simulink library "se2a_environment_lib"  (R2018b)
settings: Solver=VariableStepAuto  StartTime=0.0  StopTime=10.0  RelTol=1e-3
undefined symbols (not defined in the file or in its folder): aircraft, alt_ground, atmosphere, Atmosphere, cntrl, envir, g, ic, pos_ref, wind
libraries: simulink x9, atmosphere_lib x6, linear_systems_lib x6, $bdroot x5
(part 2 of 2)

== system se2a_environment_lib/Environment with Lidar WindEst/wind at wings1/Sort_TrueWind_Wing ==
  True_Wind_Sec : Inport
  Matrix Concatenate : Concatenate  NumInputs=3  Mode=Multidimensional array
  Matrix Concatenate1 : Concatenate  NumInputs=3  Mode=Multidimensional array
  Reshape{,1..5} (6 alike) : Reshape  OutputDimensionality=Row vector (2-D)
  u_Wg_dt_wing : Selector  InputPortWidth=6*n_wing  IndexOptions=Index vector (dialog)  Indices=(1+3*n_wing):(4*n_wing)  OutputSizes=size(Atmosphere.RequiredWindOutputs,1)-3
  u_Wg_wing : Selector  InputPortWidth=6*n_wing  IndexOptions=Index vector (dialog)  Indices=1:n_wing  OutputSizes=size(Atmosphere.RequiredWindOutputs,1)-3
  v_Wg_dt_wing : Selector  InputPortWidth=6*n_wing  IndexOptions=Index vector (dialog)  Indices=(1+4*n_wing):(5*n_wing)  OutputSizes=size(Atmosphere.RequiredWindOutputs,1)-3
  v_Wg_wing : Selector  InputPortWidth=6*n_wing  IndexOptions=Index vector (dialog)  Indices=(1+n_wing):(2*n_wing)  OutputSizes=size(Atmosphere.RequiredWindOutputs,1)-3
  w_Wg_dt_wing : Selector  InputPortWidth=6*n_wing  IndexOptions=Index vector (dialog)  Indices=(1+5*n_wing):(6*n_wing)  OutputSizes=size(Atmosphere.RequiredWindOutputs,1)-3
  w_Wg_wing : Selector  InputPortWidth=6*n_wing  IndexOptions=Index vector (dialog)  Indices=(1+2*n_wing):(3*n_wing)  OutputSizes=size(Atmosphere.RequiredWindOutputs,1)-3
  V_Wg : Outport
  V_Wg_dt : Outport  Port=2
  wires:
  v_Wg_dt_wing/1 -> Reshape4/1
  Reshape3/1 -> Matrix Concatenate1/1
  True_Wind_Sec/1 -> v_Wg_wing/1, u_Wg_wing/1, w_Wg_wing/1, w_Wg_dt_wing/1, v_Wg_dt_wing/1, u_Wg_dt_wing/1
  w_Wg_dt_wing/1 -> Reshape5/1
  Reshape/1 -> Matrix Concatenate/1
  w_Wg_wing/1 -> Reshape2/1
  v_Wg_wing/1 -> Reshape1/1
  Reshape1/1 -> Matrix Concatenate/2
  u_Wg_wing/1 -> Reshape/1
  Reshape4/1 -> Matrix Concatenate1/2
  Reshape2/1 -> Matrix Concatenate/3
  Reshape5/1 -> Matrix Concatenate1/3
  u_Wg_dt_wing/1 -> Reshape3/1
  Matrix Concatenate1/1 -> V_Wg_dt/1
  Matrix Concatenate/1 -> V_Wg/1

== system se2a_environment_lib/Environment with Lidar WindEst/wind at wings1/Sort_TrueWind_Wing1 ==
  True_Wind_Sec : Inport
  Matrix Concatenate : Concatenate  NumInputs=3  Mode=Multidimensional array
  Matrix Concatenate1 : Concatenate  NumInputs=3  Mode=Multidimensional array
  Reshape{,1..5} (6 alike) : Reshape  OutputDimensionality=Row vector (2-D)
  u_Wg_dt_wing : Selector  InputPortWidth=6*n_wing  IndexOptions=Index vector (dialog)  Indices=(1+3*n_wing):(4*n_wing)  OutputSizes=size(Atmosphere.RequiredWindOutputs,1)-3
  u_Wg_wing : Selector  InputPortWidth=6*n_wing  IndexOptions=Index vector (dialog)  Indices=1:n_wing  OutputSizes=size(Atmosphere.RequiredWindOutputs,1)-3
  v_Wg_dt_wing : Selector  InputPortWidth=6*n_wing  IndexOptions=Index vector (dialog)  Indices=(1+4*n_wing):(5*n_wing)  OutputSizes=size(Atmosphere.RequiredWindOutputs,1)-3
  v_Wg_wing : Selector  InputPortWidth=6*n_wing  IndexOptions=Index vector (dialog)  Indices=(1+n_wing):(2*n_wing)  OutputSizes=size(Atmosphere.RequiredWindOutputs,1)-3
  w_Wg_dt_wing : Selector  InputPortWidth=6*n_wing  IndexOptions=Index vector (dialog)  Indices=(1+5*n_wing):(6*n_wing)  OutputSizes=size(Atmosphere.RequiredWindOutputs,1)-3
  w_Wg_wing : Selector  InputPortWidth=6*n_wing  IndexOptions=Index vector (dialog)  Indices=(1+2*n_wing):(3*n_wing)  OutputSizes=size(Atmosphere.RequiredWindOutputs,1)-3
  V_Wg : Outport
  V_Wg_dt : Outport  Port=2
  wires:
  Matrix Concatenate/1 -> V_Wg/1
  Matrix Concatenate1/1 -> V_Wg_dt/1
  u_Wg_dt_wing/1 -> Reshape3/1
  Reshape5/1 -> Matrix Concatenate1/3
  Reshape2/1 -> Matrix Concatenate/3
  Reshape4/1 -> Matrix Concatenate1/2
  u_Wg_wing/1 -> Reshape/1
  Reshape1/1 -> Matrix Concatenate/2
  v_Wg_wing/1 -> Reshape1/1
  w_Wg_wing/1 -> Reshape2/1
  Reshape/1 -> Matrix Concatenate/1
  w_Wg_dt_wing/1 -> Reshape5/1
  True_Wind_Sec/1 -> u_Wg_dt_wing/1, v_Wg_dt_wing/1, w_Wg_dt_wing/1, w_Wg_wing/1, u_Wg_wing/1, v_Wg_wing/1
  Reshape3/1 -> Matrix Concatenate1/1
  v_Wg_dt_wing/1 -> Reshape4/1

== system se2a_environment_lib/Environment with Lidar WindEst/wind at wings1/Sort_TrueWind_Wing2 ==
  True_Wind_Sec : Inport
  Matrix Concatenate : Concatenate  NumInputs=3  Mode=Multidimensional array
  Matrix Concatenate1 : Concatenate  NumInputs=3  Mode=Multidimensional array
  Reshape{,1..5} (6 alike) : Reshape  OutputDimensionality=Row vector (2-D)
  u_Wg_dt_wing : Selector  InputPortWidth=6*n_wing  IndexOptions=Index vector (dialog)  Indices=(1+3*n_wing):(4*n_wing)  OutputSizes=size(Atmosphere.RequiredWindOutputs,1)-3
  u_Wg_wing : Selector  InputPortWidth=6*n_wing  IndexOptions=Index vector (dialog)  Indices=1:n_wing  OutputSizes=size(Atmosphere.RequiredWindOutputs,1)-3
  v_Wg_dt_wing : Selector  InputPortWidth=6*n_wing  IndexOptions=Index vector (dialog)  Indices=(1+4*n_wing):(5*n_wing)  OutputSizes=size(Atmosphere.RequiredWindOutputs,1)-3
  v_Wg_wing : Selector  InputPortWidth=6*n_wing  IndexOptions=Index vector (dialog)  Indices=(1+n_wing):(2*n_wing)  OutputSizes=size(Atmosphere.RequiredWindOutputs,1)-3
  w_Wg_dt_wing : Selector  InputPortWidth=6*n_wing  IndexOptions=Index vector (dialog)  Indices=(1+5*n_wing):(6*n_wing)  OutputSizes=size(Atmosphere.RequiredWindOutputs,1)-3
  w_Wg_wing : Selector  InputPortWidth=6*n_wing  IndexOptions=Index vector (dialog)  Indices=(1+2*n_wing):(3*n_wing)  OutputSizes=size(Atmosphere.RequiredWindOutputs,1)-3
  V_Wg : Outport
  V_Wg_dt : Outport  Port=2
  wires:
  v_Wg_dt_wing/1 -> Reshape4/1
  Reshape3/1 -> Matrix Concatenate1/1
  True_Wind_Sec/1 -> v_Wg_wing/1, u_Wg_wing/1, w_Wg_wing/1, w_Wg_dt_wing/1, v_Wg_dt_wing/1, u_Wg_dt_wing/1
  w_Wg_dt_wing/1 -> Reshape5/1
  Reshape/1 -> Matrix Concatenate/1
  w_Wg_wing/1 -> Reshape2/1
  v_Wg_wing/1 -> Reshape1/1
  Reshape1/1 -> Matrix Concatenate/2
  u_Wg_wing/1 -> Reshape/1
  Reshape4/1 -> Matrix Concatenate1/2
  Reshape2/1 -> Matrix Concatenate/3
  Reshape5/1 -> Matrix Concatenate1/3
  u_Wg_dt_wing/1 -> Reshape3/1
  Matrix Concatenate1/1 -> V_Wg_dt/1
  Matrix Concatenate/1 -> V_Wg/1

== system se2a_environment_lib/Environment with single external wind input/wind filter/Filter u ==
  u : Inport
  tau : Inport  Port=2
  Divide : Product  Inputs=*/
  Integrator : Integrator
  Sum : Sum  Inputs=|+-
  y : Outport
  y_dt : Outport  Port=2
  wires:
  u/1 -> Sum/1
  Integrator/1 -> Sum/2, y/1
  Divide/1 -> y_dt/1, Integrator/1
  Sum/1 -> Divide/1
  tau/1 -> Divide/2

== system se2a_environment_lib/Environment with single external wind input/wind filter/Filter v ==
  u : Inport
  tau : Inport  Port=2
  Divide : Product  Inputs=*/
  Integrator : Integrator
  Sum : Sum  Inputs=|+-
  y : Outport
  y_dt : Outport  Port=2
  wires:
  tau/1 -> Divide/2
  Sum/1 -> Divide/1
  Divide/1 -> Integrator/1, y_dt/1
  Integrator/1 -> y/1, Sum/2
  u/1 -> Sum/1

== system se2a_environment_lib/Environment with single external wind input/wind filter/Filter w ==
  u : Inport
  tau : Inport  Port=2
  Divide : Product  Inputs=*/
  Integrator : Integrator
  Sum : Sum  Inputs=|+-
  y : Outport
  y_dt : Outport  Port=2
  wires:
  u/1 -> Sum/1
  Integrator/1 -> Sum/2, y/1
  Divide/1 -> y_dt/1, Integrator/1
  Sum/1 -> Divide/1
  tau/1 -> Divide/2

== system se2a_environment_lib/Environment with zonal external wind input linear/wind filter/Filter u ==
  u : Inport
  tau : Inport  Port=2
  Divide : Product  Inputs=*/
  Integrator : Integrator
  Sum : Sum  Inputs=|+-
  y : Outport
  y_dt : Outport  Port=2
  wires:
  tau/1 -> Divide/2
  Sum/1 -> Divide/1
  Divide/1 -> Integrator/1, y_dt/1
  Integrator/1 -> y/1, Sum/2
  u/1 -> Sum/1

== system se2a_environment_lib/Environment with zonal external wind input linear/wind filter/Filter v ==
  u : Inport
  tau : Inport  Port=2
  Divide : Product  Inputs=*/
  Integrator : Integrator
  Sum : Sum  Inputs=|+-
  y : Outport
  y_dt : Outport  Port=2
  wires:
  u/1 -> Sum/1
  Integrator/1 -> Sum/2, y/1
  Divide/1 -> y_dt/1, Integrator/1
  Sum/1 -> Divide/1
  tau/1 -> Divide/2

== system se2a_environment_lib/Environment with zonal external wind input linear/wind filter/Filter w ==
  u : Inport
  tau : Inport  Port=2
  Divide : Product  Inputs=*/
  Integrator : Integrator
  Sum : Sum  Inputs=|+-
  y : Outport
  y_dt : Outport  Port=2
  wires:
  tau/1 -> Divide/2
  Sum/1 -> Divide/1
  Divide/1 -> Integrator/1, y_dt/1
  Integrator/1 -> y/1, Sum/2
  u/1 -> Sum/1

== matlab function se2a_environment_lib/Environment with single 1-cos gusts/MATLAB Function ==
  data: V_Kg input; V_K output
function V_K = fcn(V_Kg)
V_K = norm(V_Kg,2);
end

== matlab function se2a_environment_lib/Environment with successive 1-cos gusts/MATLAB Function ==
  data: V_Kg input; V_K output
function V_K = fcn(V_Kg)
V_K = norm(V_Kg,2);
end

== matlab function se2a_environment_lib/Environment with zonal external wind input linear/wind filter/MATLAB Function1 ==
  data: c_max input; k_max input; V input; T_cutoff output
function T_cutoff = fcn(c_max, k_max, V)
V = max(1,V);
omega_max = k_max * V / (c_max/2);
T_cutoff = 1/omega_max;
end

== matlab function se2a_environment_lib/Environment with single external wind input/MATLAB Function ==
  data: V_Kg input; V_K output
function V_K = fcn(V_Kg)
V_K = norm(V_Kg,2);
end

== matlab function se2a_environment_lib/Environment with zonal external wind input linear/MATLAB Function ==
  data: V_Kg input; V_K output
function V_K = fcn(V_Kg)
V_K = norm(V_Kg,2);
end

== matlab function se2a_environment_lib/Environment with single 1-cos gusts/1-cos gust generator/MATLAB Function1 ==
  data: h input; U output; gustGradDist input; F_g input; s input; U_ds output
function [U,U_ds] = fcn(h,gustGradDist,F_g,s)

% define 1-cos gust
U_ref           = oneMinusCosGustUref( h );
U_ds            = oneMinusCosGustUds( U_ref, gustGradDist, F_g );
U               = U_ds/2 * ( 1 - cos( pi*s/gustGradDist ) );

end

== matlab function se2a_environment_lib/Environment with single 1-cos gusts/1-cos gust generator/MATLAB Function2 ==
  data: gustGradDist input; gustOver output; s input; delta_time input; time_between_gusts input; noGust output; nextGust output
function [ gustOver, noGust, nextGust ] = fcn(gustGradDist, s, delta_time,time_between_gusts) %#codegen

if s >= 2*gustGradDist
    gustOver = 1;
else
    gustOver = 0;
end

if  delta_time > 0 && delta_time < time_between_gusts
    noGust = 1;
else
    noGust = 0;
end

if delta_time >= time_between_gusts
    nextGust = 1;
else
    nextGust = 0;
end

end

== matlab function se2a_environment_lib/Environment with single external wind input/wind filter/MATLAB Function1 ==
  data: c_max input; k_max input; V input; T_cutoff output
function T_cutoff = fcn(c_max, k_max, V)
V = max(1,V);
omega_max = k_max * V / (c_max/2);
T_cutoff = 1/omega_max;
end

== matlab function se2a_environment_lib/Environment with single 1-cos gusts/1-cos gust generator/MATLAB Function3 ==
  data: gustGradDist_old input; increment input; gustGradDist output; gustOver input
function gustGradDist = fcn( gustGradDist_old, increment, gustOver ) %#codegen

if gustOver
    gustGradDist = gustGradDist_old + increment;
else
    gustGradDist = gustGradDist_old;
end

== matlab function se2a_environment_lib/Environment with single 1-cos gusts/1-cos gust generator/ft2m ==
  data: u input; y output
function y = fcn(u)
y = ft2m(u);
